simulink subsystem "sensores"  (R2023b)
settings: Solver=VariableStepAuto  StartTime=0.0  StopTime=10.0  RelTol=1e-3
settings Model: Creator=rodri  LastModifiedBy=nahue

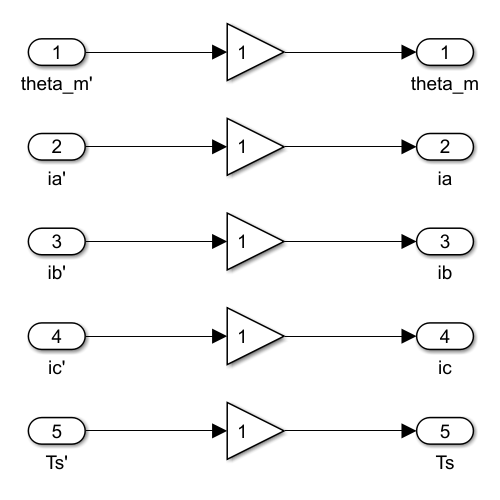
[thumbnail: Simulink's stored preview of the top-level diagram]
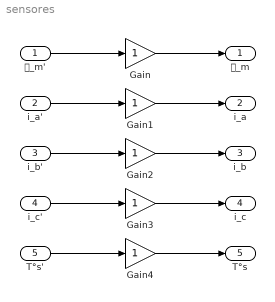
== system sensores ==
  𝜃_m' : Inport
  i_a' : Inport  Port=2
  i_b' : Inport  Port=3
  i_c' : Inport  Port=4
  T°s' : Inport  Port=5
  Gain{,1..4} (5 alike) : Gain
  𝜃_m : Outport
  i_a : Outport  Port=2
  i_b : Outport  Port=3
  i_c : Outport  Port=4
  T°s : Outport  Port=5
  wires:
  𝜃_m'/1 -> Gain/1
  Gain/1 -> 𝜃_m/1
  i_a'/1 -> Gain1/1
  Gain1/1 -> i_a/1
  i_b'/1 -> Gain2/1
  Gain2/1 -> i_b/1
  i_c'/1 -> Gain3/1
  Gain3/1 -> i_c/1
  T°s'/1 -> Gain4/1
  Gain4/1 -> T°s/1
